simulink library "lookUpTotalGaitDynamics"  (R2016b)
settings: Solver=VariableStepAuto  StartTime=0.0  StopTime=10.0  RelTol=1e-3
libraries: lookUpGaitDynamics x4, VariousLibrary x1
settings Model: Creator=march  LastModifiedBy=Taeke

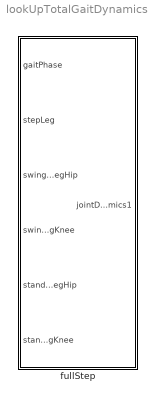
== system lookUpTotalGaitDynamics ==
  fullStep : Subsystem

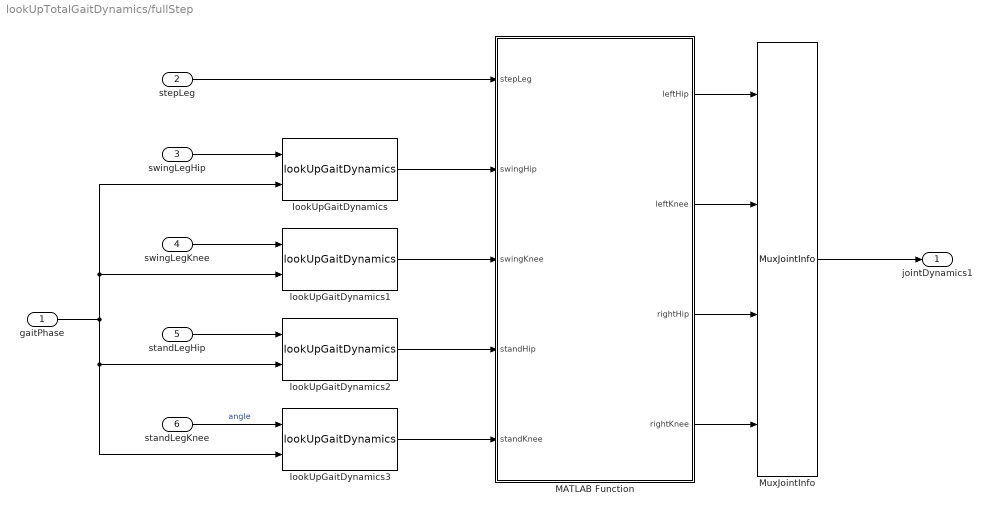
== system lookUpTotalGaitDynamics/fullStep ==
  gaitPhase : Inport
  stepLeg : Inport  Port=2
  swingLegHip : Inport  Port=3
  swingLegKnee : Inport  Port=4
  standLegHip : Inport  Port=5
  standLegKnee : Inport  Port=6
  MATLAB Function : MATLAB Function  TreatAsAtomicUnit=on
  MuxJointInfo : VariousLibrary/MuxJointInfo
  lookUpGaitDynamics{,1..3} (4 alike) : lookUpGaitDynamics/lookUpGaitDynamics
  jointDynamics1 : Outport  OutDataTypeStr=Bus: JointDynamics
  wires:
  MATLAB Function/4(rightKnee) -> MuxJointInfo/4
  MATLAB Function/3(rightHip) -> MuxJointInfo/3
  MATLAB Function/2(leftKnee) -> MuxJointInfo/2
  MATLAB Function/1(leftHip) -> MuxJointInfo/1
  lookUpGaitDynamics3/1 -> MATLAB Function/5(standKnee)
  lookUpGaitDynamics2/1 -> MATLAB Function/4(standHip)
  lookUpGaitDynamics1/1 -> MATLAB Function/3(swingKnee)
  lookUpGaitDynamics/1 -> MATLAB Function/2(swingHip)
  stepLeg/1 -> MATLAB Function/1(stepLeg)
  swingLegHip/1 -> lookUpGaitDynamics/1
  swingLegKnee/1 -> lookUpGaitDynamics1/1
  standLegKnee/1 -> lookUpGaitDynamics3/1  "angle"
  standLegHip/1 -> lookUpGaitDynamics2/1
  gaitPhase/1 -> lookUpGaitDynamics/2, lookUpGaitDynamics1/2, lookUpGaitDynamics2/2, lookUpGaitDynamics3/2
  MuxJointInfo/1 -> jointDynamics1/1

== matlab function lookUpTotalGaitDynamics/fullStep/MATLAB Function ==
  data: stepLeg input; leftHip output Bus: JointDynamics; swingHip input Bus: JointDynamics; swingKnee input Bus: JointDynamics; standHip input Bus: JointDynamics; standKnee input Bus: JointDynamics; leftKnee output Bus: JointDynamics; rightHip output Bus: JointDynamics; rightKnee output Bus: JointDynamics
function [ leftHip, leftKnee, rightHip, rightKnee ] = routeSwingToLeg(stepLeg, swingHip, swingKnee, standHip, standKnee )
% wrapper for routeSwingToLeg
[ leftHip, leftKnee, rightHip, rightKnee ] = routeSwingToLeg(stepLeg, swingHip, swingKnee, standHip, standKnee );
end
